simulink model "CoPT_TrqLeadCoord"  (R2016b)
settings: configuration reference "CodeGenConfigSet" (kept outside this file)
values from neighbouring files (symbols this model uses):
  CoPT_dtrqCurrCorP_Neg_C = Calibration.Parameter    [init_CoPT_TrqLeadCoord.m]    (also in init_CoPT_TrqLeadCoord_SIL.m = Simulink.Parameter)
  CoPT_dtrqCurrCorP_Pos_C = Calibration.Parameter    [init_CoPT_TrqLeadCoord.m]    (also in init_CoPT_TrqLeadCoord_SIL.m = Simulink.Parameter)
  CoPT_tiDebCurr_C = Calibration.Parameter    [init_CoPT_TrqLeadCoord.m]    (also in init_CoPT_TrqLeadCoord_SIL.m = Simulink.Parameter)
  CoPT_tiDebLead_C = Calibration.Parameter    [init_CoPT_TrqLeadCoord.m]    (also in init_CoPT_TrqLeadCoord_SIL.m = Simulink.Parameter)
  DFFTLPRT_OVRDS_TSCINC = fi(1,State_int32)    [init_CoPT_TrqLeadCoord.m]    (also in init_CoPT_TrqLeadCoord_SIL.m)
  DFFTLPRTOVRDSTSCINC_SY = fi(1,State_int32)    [init_CoPT_TrqLeadCoord.m]    (also in init_CoPT_TrqLeadCoord_SIL.m)
undefined symbols (not defined in the file or in its folder): CoPT_TrqLeadCoord_DT
libraries: CXLib x8
settings Model: Creator=Wollf  LastModifiedBy=bianxuyin
settings ConfigSetRef: SourceLocation=Base Workspace

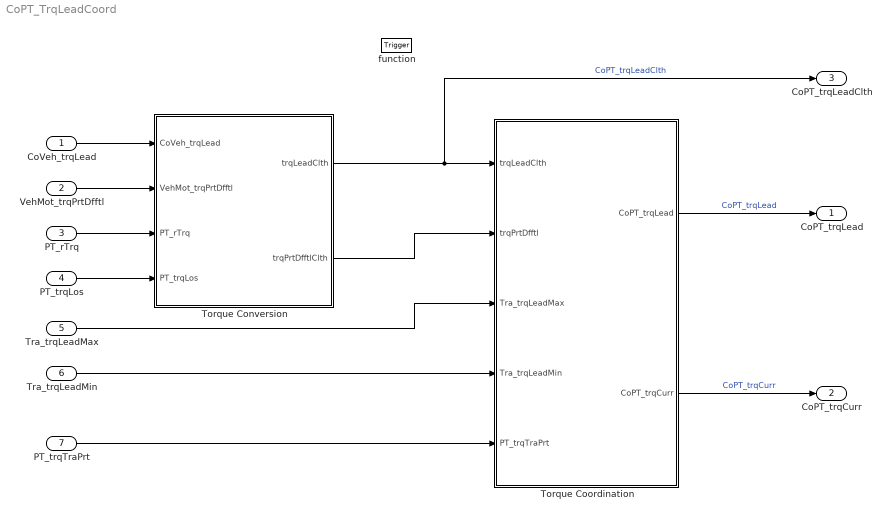
== system CoPT_TrqLeadCoord ==
  CoVeh_trqLead : Inport  Tag=Nm  Description=Lead torque order on the drive train (gearbox output torque)  OutMin=-3000  OutMax=3000  OutDataTypeStr=Trq_Nm
  VehMot_trqPrtDfftl : Inport  Tag=Nm  Description=Differential protection torque  Port=2  OutMin=-3000  OutMax=3000  OutDataTypeStr=Trq_Nm
  PT_rTrq : Inport  Description=Powertrain torque ratio  Port=3  OutMin=-100  OutMax=100  OutDataTypeStr=TransRatio
  PT_trqLos : Inport  Tag=Nm  Description=Parameter for loss torque of the drive train  Port=4  OutMin=-3000  OutMax=3000  OutDataTypeStr=Trq_Nm
  Tra_trqLeadMax : Inport  Tag=Nm  Description=decrement lead torque demand from gearbox  Port=5  OutMin=-3000  OutMax=3000  OutDataTypeStr=Trq_Nm
  Tra_trqLeadMin : Inport  Tag=Nm  Description=increment lead torque demand from gearbox  Port=6  OutMin=-3000  OutMax=3000  OutDataTypeStr=Trq_Nm
  PT_trqTraPrt : Inport  Tag=Nm  Description=Maximum allowed inner torque  Port=7  OutMin=-3000  OutMax=3000  OutDataTypeStr=Trq_Nm
  function : TriggerPort  TriggerType=function-call  VariantControl=Variant
  Torque Conversion : Subsystem
  Torque Coordination : Subsystem
  CoPT_trqLead : Outport  Tag=Nm  Description=Rate action moment order moment place (Clutch moment)  OutMin=-3000  OutMax=3000  OutDataTypeStr=Trq_Nm
  CoPT_trqCurr : Outport  Tag=Nm  Description=Lead torque order for rail pressure control (clutch torque)  Port=2  OutMin=-3000  OutMax=3000  OutDataTypeStr=Trq_Nm
  CoPT_trqLeadClth : Outport  Tag=Nm  Description=Lead torque demand at gearbox  Port=3  OutMin=-3000  OutMax=3000  OutDataTypeStr=Trq_Nm
  wires:
  Torque Conversion/1(trqLeadClth) -> CoPT_trqLeadClth/1, Torque Coordination/1(trqLeadClth)  "CoPT_trqLeadClth"
  Torque Conversion/2(trqPrtDfftlClth) -> Torque Coordination/2(trqPrtDfftl)
  PT_trqLos/1 -> Torque Conversion/4(PT_trqLos)
  PT_rTrq/1 -> Torque Conversion/3(PT_rTrq)
  VehMot_trqPrtDfftl/1 -> Torque Conversion/2(VehMot_trqPrtDfftl)
  CoVeh_trqLead/1 -> Torque Conversion/1(CoVeh_trqLead)
  Tra_trqLeadMax/1 -> Torque Coordination/3(Tra_trqLeadMax)
  PT_trqTraPrt/1 -> Torque Coordination/5(PT_trqTraPrt)
  Torque Coordination/2(CoPT_trqCurr) -> CoPT_trqCurr/1  "CoPT_trqCurr"
  Tra_trqLeadMin/1 -> Torque Coordination/4(Tra_trqLeadMin)
  Torque Coordination/1(CoPT_trqLead) -> CoPT_trqLead/1  "CoPT_trqLead"

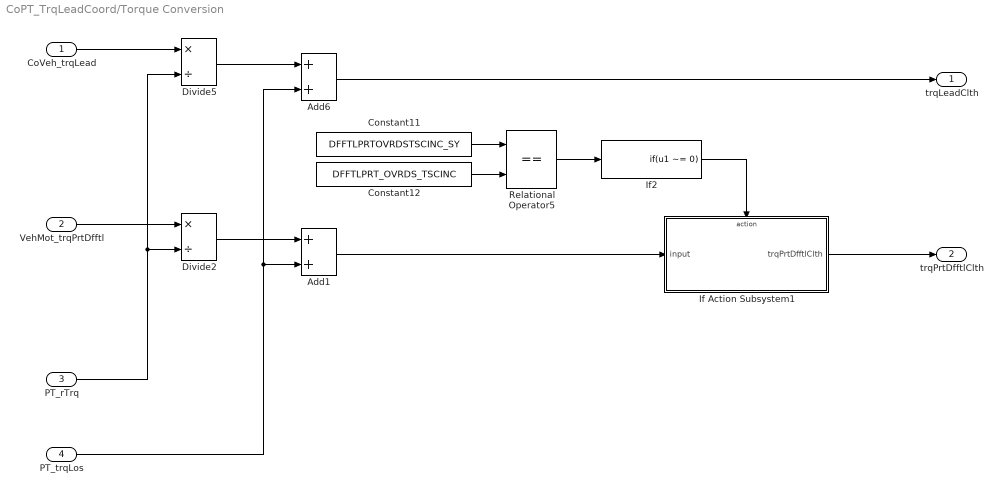
== system CoPT_TrqLeadCoord/Torque Conversion ==
  CoVeh_trqLead : Inport
  VehMot_trqPrtDfftl : Inport  Port=2
  PT_rTrq : Inport  Port=3
  PT_trqLos : Inport  Port=4
  Add1 : Sum  SaturateOnIntegerOverflow=on  InputSameDT=on
  Add6 : Sum  SaturateOnIntegerOverflow=on  InputSameDT=on
  Constant11 : Constant  Value=DFFTLPRTOVRDSTSCINC_SY
  Constant12 : Constant  Value=DFFTLPRT_OVRDS_TSCINC
  Divide2 : Product  Inputs=*/  OutDataTypeStr=Trq_Nm  SaturateOnIntegerOverflow=on
  Divide5 : Product  Inputs=*/  OutDataTypeStr=Trq_Nm  SaturateOnIntegerOverflow=on
  If Action Subsystem1 : Subsystem  TreatAsAtomicUnit=on
  If2 : If  IfExpression=u1 ~= 0  ShowElse=off
  Relational Operator5 : RelationalOperator  Operator===  OutDataTypeStr=boolean  RndMeth=Simplest  InputSameDT=on
  trqLeadClth : Outport
  trqPrtDfftlClth : Outport  Port=2
  wires:
  PT_rTrq/1 -> Divide5/2, Divide2/2
  CoVeh_trqLead/1 -> Divide5/1
  PT_trqLos/1 -> Add6/2, Add1/2
  Add6/1 -> trqLeadClth/1
  Divide5/1 -> Add6/1
  Add1/1 -> If Action Subsystem1/1(input)
  Constant11/1 -> Relational Operator5/1
  Relational Operator5/1 -> If2/1
  If2/1 -> If Action Subsystem1/Action
  Divide2/1 -> Add1/1
  Constant12/1 -> Relational Operator5/2
  VehMot_trqPrtDfftl/1 -> Divide2/1
  If Action Subsystem1/1(trqPrtDfftlClth) -> trqPrtDfftlClth/1

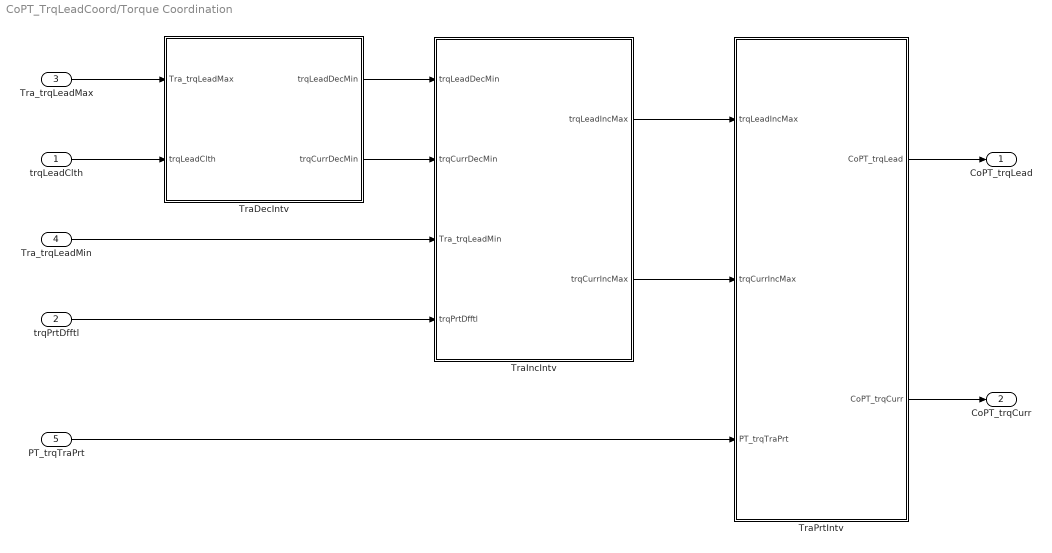
== system CoPT_TrqLeadCoord/Torque Coordination ==
  trqLeadClth : Inport
  trqPrtDfftl : Inport  Port=2
  Tra_trqLeadMax : Inport  Port=3
  Tra_trqLeadMin : Inport  Port=4
  PT_trqTraPrt : Inport  Port=5
  TraDecIntv : Subsystem
  TraIncIntv : Subsystem
  TraPrtIntv : Subsystem
  CoPT_trqLead : Outport
  CoPT_trqCurr : Outport  Port=2
  wires:
  TraPrtIntv/2(CoPT_trqCurr) -> CoPT_trqCurr/1
  TraPrtIntv/1(CoPT_trqLead) -> CoPT_trqLead/1
  PT_trqTraPrt/1 -> TraPrtIntv/3(PT_trqTraPrt)
  TraDecIntv/2(trqCurrDecMin) -> TraIncIntv/2(trqCurrDecMin)
  TraDecIntv/1(trqLeadDecMin) -> TraIncIntv/1(trqLeadDecMin)
  trqPrtDfftl/1 -> TraIncIntv/4(trqPrtDfftl)
  Tra_trqLeadMin/1 -> TraIncIntv/3(Tra_trqLeadMin)
  TraIncIntv/2(trqCurrIncMax) -> TraPrtIntv/2(trqCurrIncMax)
  trqLeadClth/1 -> TraDecIntv/2(trqLeadClth)
  Tra_trqLeadMax/1 -> TraDecIntv/1(Tra_trqLeadMax)
  TraIncIntv/1(trqLeadIncMax) -> TraPrtIntv/1(trqLeadIncMax)

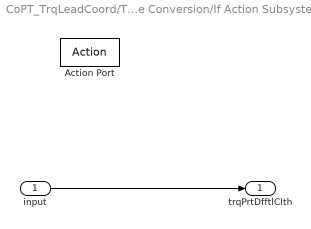
== system CoPT_TrqLeadCoord/Torque Conversion/If Action Subsystem1 ==
  input : Inport
  Action Port : ActionPort  ActionType=then
  trqPrtDfftlClth : Outport
  wires:
  input/1 -> trqPrtDfftlClth/1

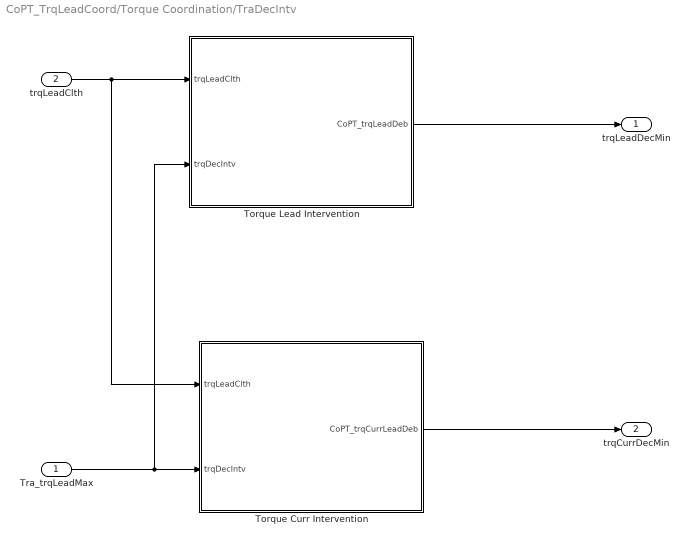
== system CoPT_TrqLeadCoord/Torque Coordination/TraDecIntv ==
  Tra_trqLeadMax : Inport
  trqLeadClth : Inport  Port=2
  Torque Curr Intervention : Subsystem
  Torque Lead Intervention : Subsystem
  trqLeadDecMin : Outport
  trqCurrDecMin : Outport  Port=2
  wires:
  Tra_trqLeadMax/1 -> Torque Lead Intervention/2(trqDecIntv), Torque Curr Intervention/2(trqDecIntv)
  Torque Curr Intervention/1(CoPT_trqCurrLeadDeb) -> trqCurrDecMin/1
  trqLeadClth/1 -> Torque Curr Intervention/1(trqLeadClth), Torque Lead Intervention/1(trqLeadClth)
  Torque Lead Intervention/1(CoPT_trqLeadDeb) -> trqLeadDecMin/1

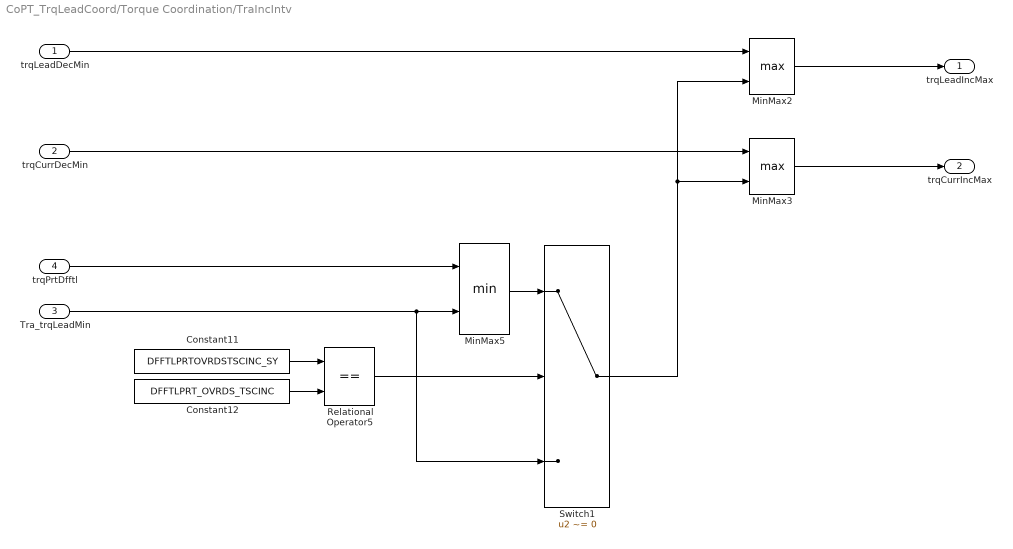
== system CoPT_TrqLeadCoord/Torque Coordination/TraIncIntv ==
  trqLeadDecMin : Inport
  trqCurrDecMin : Inport  Port=2
  Tra_trqLeadMin : Inport  Port=3
  trqPrtDfftl : Inport  Port=4
  Constant11 : Constant  Value=DFFTLPRTOVRDSTSCINC_SY
  Constant12 : Constant  Value=DFFTLPRT_OVRDS_TSCINC
  MinMax2 : MinMax  Function=max  Inputs=2  InputSameDT=on
  MinMax3 : MinMax  Function=max  Inputs=2  InputSameDT=on
  MinMax5 : MinMax  Inputs=2  InputSameDT=on
  Relational Operator5 : RelationalOperator  Operator===  OutDataTypeStr=boolean  RndMeth=Simplest  InputSameDT=on
  Switch1 : Switch  Criteria=u2 ~= 0  InputSameDT=on
  trqLeadIncMax : Outport
  trqCurrIncMax : Outport  Port=2
  wires:
  trqPrtDfftl/1 -> MinMax5/1
  Switch1/1 -> MinMax3/2, MinMax2/2
  Constant11/1 -> Relational Operator5/1
  Relational Operator5/1 -> Switch1/2
  Constant12/1 -> Relational Operator5/2
  MinMax3/1 -> trqCurrIncMax/1
  trqCurrDecMin/1 -> MinMax3/1
  MinMax5/1 -> Switch1/1
  Tra_trqLeadMin/1 -> Switch1/3, MinMax5/2
  MinMax2/1 -> trqLeadIncMax/1
  trqLeadDecMin/1 -> MinMax2/1

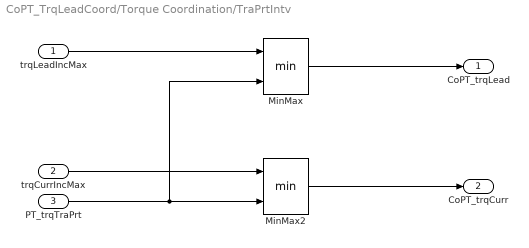
== system CoPT_TrqLeadCoord/Torque Coordination/TraPrtIntv ==
  trqLeadIncMax : Inport
  trqCurrIncMax : Inport  Port=2
  PT_trqTraPrt : Inport  Port=3
  MinMax : MinMax  Inputs=2  InputSameDT=on
  MinMax2 : MinMax  Inputs=2  InputSameDT=on
  CoPT_trqLead : Outport
  CoPT_trqCurr : Outport  Port=2
  wires:
  MinMax/1 -> CoPT_trqLead/1
  PT_trqTraPrt/1 -> MinMax/2, MinMax2/2
  trqCurrIncMax/1 -> MinMax2/1
  MinMax2/1 -> CoPT_trqCurr/1
  trqLeadIncMax/1 -> MinMax/1

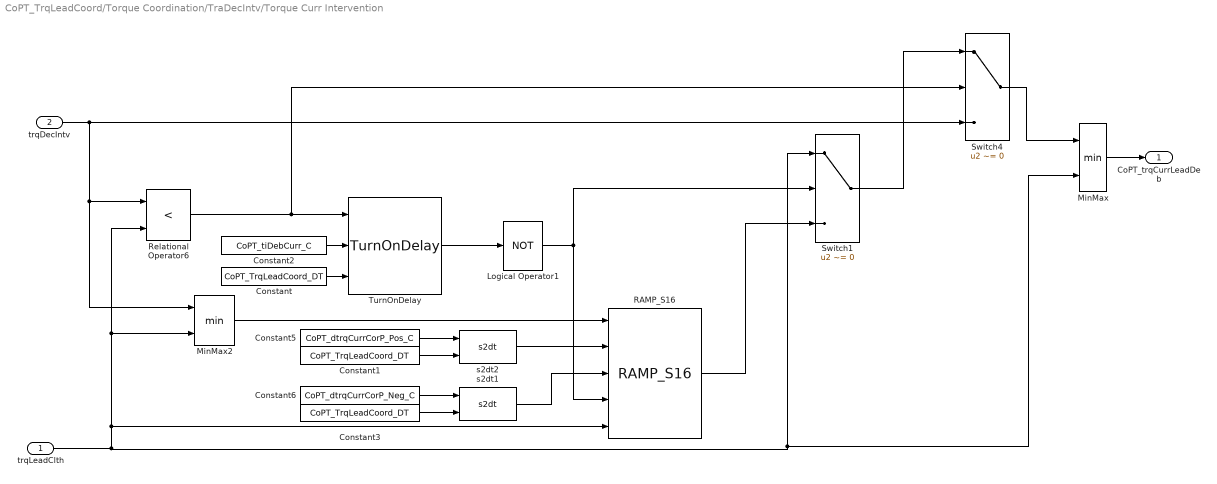
== system CoPT_TrqLeadCoord/Torque Coordination/TraDecIntv/Torque Curr Intervention ==
  trqLeadClth : Inport
  trqDecIntv : Inport  Port=2
  Constant : Constant  Value=CoPT_TrqLeadCoord_DT  OutDataTypeStr=Inherit: Inherit via back propagation
  Constant1 : Constant  Value=CoPT_TrqLeadCoord_DT  OutDataTypeStr=Inherit: Inherit via back propagation
  Constant2 : Constant  Value=CoPT_tiDebCurr_C  SampleTime=-1
  Constant3 : Constant  Value=CoPT_TrqLeadCoord_DT  OutDataTypeStr=Inherit: Inherit via back propagation
  Constant5 : Constant  Value=CoPT_dtrqCurrCorP_Pos_C
  Constant6 : Constant  Value=CoPT_dtrqCurrCorP_Neg_C
  Logical Operator1 : Logic  Operator=NOT  AllPortsSameDT=off  OutDataTypeStr=boolean
  MinMax : MinMax  Inputs=2
  MinMax2 : MinMax  Inputs=2  InputSameDT=on
  RAMP_S16 : CXLib/RAMP_S16
  Relational Operator6 : RelationalOperator  Operator=<  OutDataTypeStr=boolean  RndMeth=Simplest  InputSameDT=on
  Switch1 : Switch  Criteria=u2 ~= 0  InputSameDT=on
  Switch4 : Switch  Criteria=u2 ~= 0  InputSameDT=on
  TurnOnDelay : CXLib/TurnOnDelay
  s2dt1 : CXLib/s2dt
  s2dt2 : CXLib/s2dt
  CoPT_trqCurrLeadDeb : Outport
  wires:
  Constant/1 -> TurnOnDelay/3
  MinMax2/1 -> RAMP_S16/1
  TurnOnDelay/1 -> Logical Operator1/1
  s2dt1/1 -> RAMP_S16/3
  trqLeadClth/1 -> Relational Operator6/2, MinMax2/2, RAMP_S16/5, MinMax/2, Switch1/1
  s2dt2/1 -> RAMP_S16/2
  Relational Operator6/1 -> TurnOnDelay/1, Switch4/2
  Constant2/1 -> TurnOnDelay/2
  Logical Operator1/1 -> Switch1/2, RAMP_S16/4
  Switch1/1 -> Switch4/1
  RAMP_S16/1 -> Switch1/3
  trqDecIntv/1 -> Relational Operator6/1, MinMax2/1, Switch4/3
  Switch4/1 -> MinMax/1
  MinMax/1 -> CoPT_trqCurrLeadDeb/1
  Constant5/1 -> s2dt2/1
  Constant1/1 -> s2dt2/2
  Constant3/1 -> s2dt1/2
  Constant6/1 -> s2dt1/1

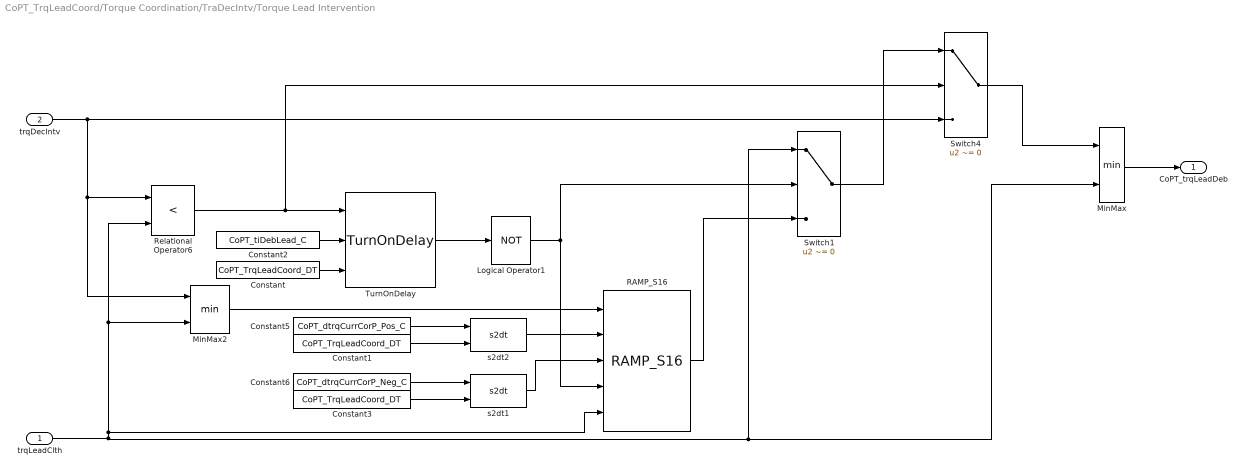
== system CoPT_TrqLeadCoord/Torque Coordination/TraDecIntv/Torque Lead Intervention ==
  trqLeadClth : Inport
  trqDecIntv : Inport  Port=2
  Constant : Constant  Value=CoPT_TrqLeadCoord_DT  OutDataTypeStr=Inherit: Inherit via back propagation
  Constant1 : Constant  Value=CoPT_TrqLeadCoord_DT  OutDataTypeStr=Inherit: Inherit via back propagation
  Constant2 : Constant  Value=CoPT_tiDebLead_C
  Constant3 : Constant  Value=CoPT_TrqLeadCoord_DT  OutDataTypeStr=Inherit: Inherit via back propagation
  Constant5 : Constant  Value=CoPT_dtrqCurrCorP_Pos_C
  Constant6 : Constant  Value=CoPT_dtrqCurrCorP_Neg_C
  Logical Operator1 : Logic  Operator=NOT  AllPortsSameDT=off  OutDataTypeStr=boolean
  MinMax : MinMax  Inputs=2
  MinMax2 : MinMax  Inputs=2  InputSameDT=on
  RAMP_S16 : CXLib/RAMP_S16
  Relational Operator6 : RelationalOperator  Operator=<  OutDataTypeStr=boolean  RndMeth=Simplest  InputSameDT=on
  Switch1 : Switch  Criteria=u2 ~= 0  InputSameDT=on
  Switch4 : Switch  Criteria=u2 ~= 0  InputSameDT=on
  TurnOnDelay : CXLib/TurnOnDelay
  s2dt1 : CXLib/s2dt
  s2dt2 : CXLib/s2dt
  CoPT_trqLeadDeb : Outport
  wires:
  Constant/1 -> TurnOnDelay/3
  trqDecIntv/1 -> Switch4/3, MinMax2/1, Relational Operator6/1
  RAMP_S16/1 -> Switch1/3
  Switch1/1 -> Switch4/1
  Logical Operator1/1 -> Switch1/2, RAMP_S16/4
  Constant2/1 -> TurnOnDelay/2
  Relational Operator6/1 -> Switch4/2, TurnOnDelay/1
  s2dt2/1 -> RAMP_S16/2
  trqLeadClth/1 -> Relational Operator6/2, MinMax2/2, RAMP_S16/5, MinMax/2, Switch1/1
  s2dt1/1 -> RAMP_S16/3
  TurnOnDelay/1 -> Logical Operator1/1
  MinMax2/1 -> RAMP_S16/1
  Switch4/1 -> MinMax/1
  MinMax/1 -> CoPT_trqLeadDeb/1
  Constant5/1 -> s2dt2/1
  Constant1/1 -> s2dt2/2
  Constant3/1 -> s2dt1/2
  Constant6/1 -> s2dt1/1
